simulink model "vessel_model"  (R2020a)
settings: Solver=FixedStepAuto  StartTime=0.0  StopTime=10  FixedStep=0.01  RelTol=1e-3
PreLoadFcn:
  | load("interfaces.mat");
libraries: simulink_extras x5
settings Model: Creator=thomas.evang  LastModifiedBy=thomas.evang
settings SFSimCC: CustomCodeUndefinedFunction=UseInterfaceOnly
settings RTWCC: Description=Generic Real-Time Target  RetainRTWFile=on

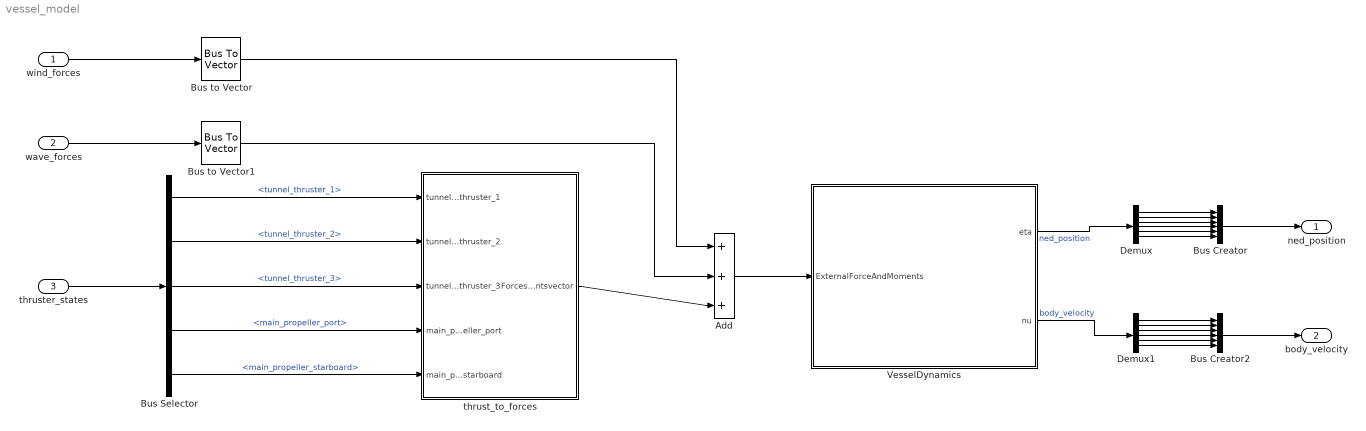
== system vessel_model ==
  wind_forces : Inport  OutDataTypeStr=Bus: force_6dof
  wave_forces : Inport  Port=2  OutDataTypeStr=Bus: force_6dof
  thruster_states : Inport  Port=3  OutDataTypeStr=Bus: thruster_states
  Add : Sum  Inputs=+++|
  Bus Creator : BusCreator  Inputs=6  OutDataTypeStr=Bus: position_6dof
      settings: InheritFromInputs=off
  Bus Creator2 : BusCreator  Inputs=6  OutDataTypeStr=Bus: velocity_6dof
      settings: InheritFromInputs=off
  Bus Selector : BusSelector  OutputSignals=tunnel_thruster_1,tunnel_thruster_2,tunnel_thruster_3,main_propeller_port,main_propeller_starboard
  Bus to Vector : BusToVector
  Bus to Vector1 : BusToVector
  Demux : Demux  Outputs=6
  Demux1 : Demux  Outputs=6
  VesselDynamics : Subsystem
  thrust_to_forces : Subsystem
  ned_position : Outport  OutDataTypeStr=Bus: position_6dof  VectorParamsAs1DForOutWhenUnconnected=off
  body_velocity : Outport  Port=2  OutDataTypeStr=Bus: velocity_6dof  VectorParamsAs1DForOutWhenUnconnected=off
  wires:
  wave_forces/1 -> Bus to Vector1/1
  wind_forces/1 -> Bus to Vector/1
  thruster_states/1 -> Bus Selector/1
  Bus Selector/1 -> thrust_to_forces/1(tunnel_thruster_1)  "<tunnel_thruster_1>"
  Bus Selector/2 -> thrust_to_forces/2(tunnel_thruster_2)  "<tunnel_thruster_2>"
  Bus Selector/3 -> thrust_to_forces/3(tunnel_thruster_3)  "<tunnel_thruster_3>"
  Bus Selector/4 -> thrust_to_forces/4(main_propeller_port)  "<main_propeller_port>"
  Bus Selector/5 -> thrust_to_forces/5(main_propeller_starboard)  "<main_propeller_starboard>"
  Bus to Vector/1 -> Add/1
  Bus to Vector1/1 -> Add/2
  VesselDynamics/1(eta) -> Demux/1  "ned_position"
  Demux/1 -> Bus Creator/1
  Demux/2 -> Bus Creator/2
  Demux/3 -> Bus Creator/3
  Demux/4 -> Bus Creator/4
  Demux/5 -> Bus Creator/5
  Demux/6 -> Bus Creator/6
  Demux1/3 -> Bus Creator2/3
  Demux1/6 -> Bus Creator2/6
  Demux1/2 -> Bus Creator2/2
  Demux1/5 -> Bus Creator2/5
  Demux1/1 -> Bus Creator2/1
  VesselDynamics/2(nu) -> Demux1/1  "body_velocity"
  Demux1/4 -> Bus Creator2/4
  Bus Creator/1 -> ned_position/1
  Bus Creator2/1 -> body_velocity/1
  thrust_to_forces/1(ForcesAndMomentsvector) -> Add/3
  Add/1 -> VesselDynamics/1(ExternalForceAndMoments)

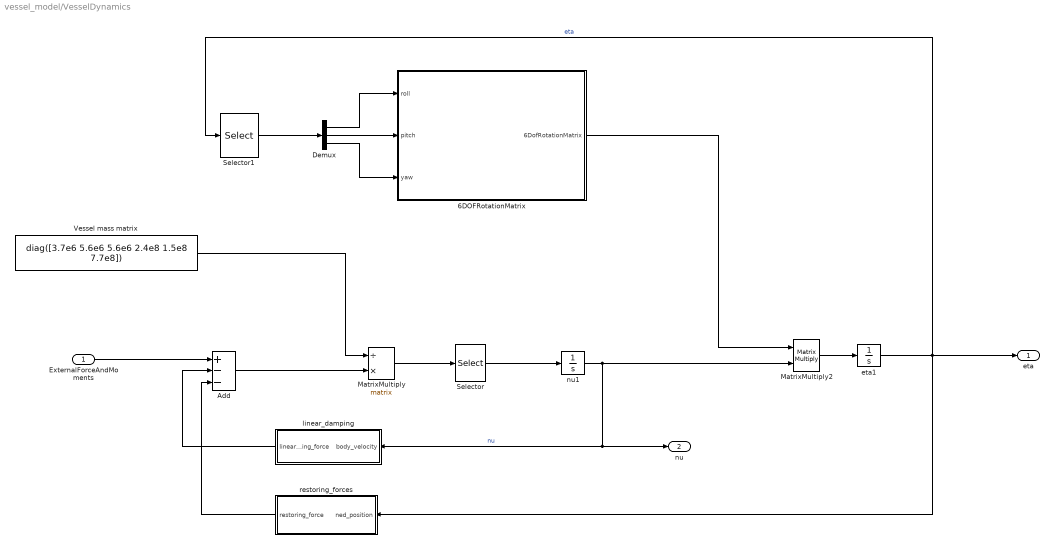
== system vessel_model/VesselDynamics ==
  ExternalForceAndMoments : Inport
  6DOFRotationMatrix : Subsystem
  Add : Sum  Inputs=+--
  Demux : Demux  Outputs=3
  MatrixMultiply : Product  Inputs=/*  Multiplication=Matrix(*)
  MatrixMultiply2 : Product  Inputs=**  Multiplication=Matrix(*)
  Selector : Selector  NumberOfDimensions=2  InputPortWidth=3  IndexOptions=Select all,Index vector (dialog)  Indices=[1 3],1  OutputSizes=1,1
  Selector1 : Selector  InputPortWidth=6  IndexOptions=Index vector (dialog)  Indices=[4 5 6]  OutputSizes=1
  Vessel mass matrix : Constant  Value=diag([3.7e6 5.6e6 5.6e6 2.4e8 1.5e8 7.7e8])
  eta1 : Integrator  InitialCondition=zeros(6,1)  ContinuousStateAttributes='nu'
  linear_damping : Subsystem
  nu1 : Integrator  InitialCondition=zeros(6,1)  ContinuousStateAttributes='eta'
  restoring_forces : Subsystem  mask{a_wp=1548, gm_t=1.5, gm_l=61, rho_w=1025, g=9.81, disp=2000*10}
      mask prompts: a_wp "Water Plane Area"; gm_t "Transverse Metacentric Height"; gm_l "Longitudal Metacentric Height"; rho_w "Density of Water"; g "Gravity"; disp "Displacement"
  eta : Outport  VectorParamsAs1DForOutWhenUnconnected=off
  nu : Outport  Port=2  VectorParamsAs1DForOutWhenUnconnected=off
  wires:
  Demux/2 -> 6DOFRotationMatrix/2(pitch)
  nu1/1 -> MatrixMultiply2/2, linear_damping/1(body_velocity), nu/1  "nu"
  Vessel mass matrix/1 -> MatrixMultiply/1
  Demux/1 -> 6DOFRotationMatrix/1(roll)
  Selector1/1 -> Demux/1
  Demux/3 -> 6DOFRotationMatrix/3(yaw)
  Add/1 -> MatrixMultiply/2
  MatrixMultiply/1 -> Selector/1
  Selector/1 -> nu1/1
  6DOFRotationMatrix/1(6DofRotationMatrix) -> MatrixMultiply2/1
  eta1/1 -> eta/1, restoring_forces/1(ned_position), Selector1/1  "eta"
  ExternalForceAndMoments/1 -> Add/1
  MatrixMultiply2/1 -> eta1/1
  restoring_forces/1(restoring_force) -> Add/3
  linear_damping/1(linear_damping_force) -> Add/2

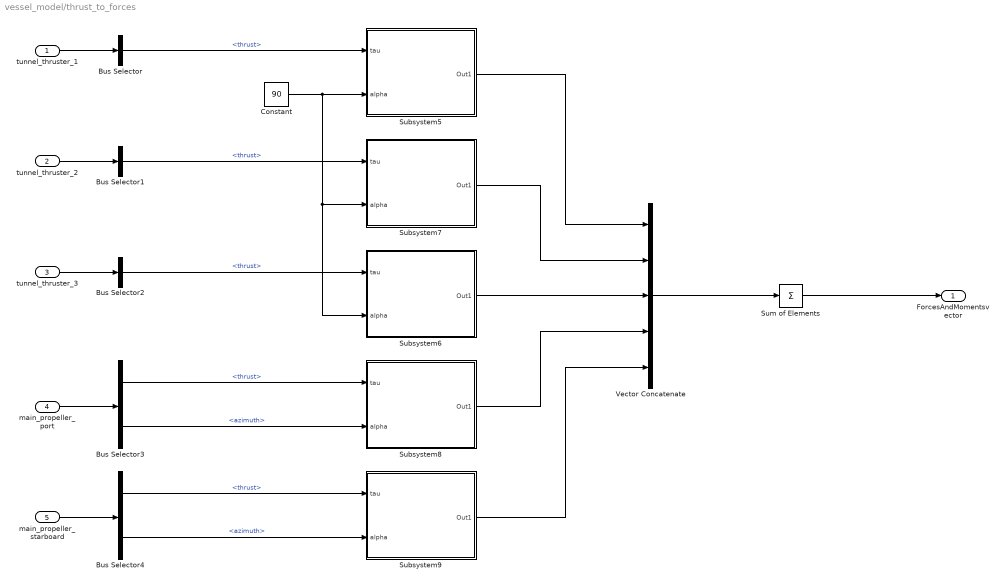
== system vessel_model/thrust_to_forces ==
  tunnel_thruster_1 : Inport  OutDataTypeStr=Bus: tunnel_thruster
  tunnel_thruster_2 : Inport  Port=2  OutDataTypeStr=Bus: tunnel_thruster
  tunnel_thruster_3 : Inport  Port=3  OutDataTypeStr=Bus: tunnel_thruster
  main_propeller_port : Inport  Port=4  OutDataTypeStr=Bus: azimuth_thruster
  main_propeller_starboard : Inport  Port=5  OutDataTypeStr=Bus: azimuth_thruster
  Bus Selector : BusSelector  OutputSignals=thrust
  Bus Selector1 : BusSelector  OutputSignals=thrust
  Bus Selector2 : BusSelector  OutputSignals=thrust
  Bus Selector3 : BusSelector  OutputSignals=thrust,azimuth
  Bus Selector4 : BusSelector  OutputSignals=thrust,azimuth
  Constant : Constant  Value=90
  Subsystem5 : Subsystem  mask{x=31.25, y=0, z=2.1}
  Subsystem6 : Subsystem  mask{x=24.75, y=0, z=1.9}
  Subsystem7 : Subsystem  mask{x=28.9, y=0, z=1.9}
  Subsystem8 : Subsystem  mask{x=-36.45, y=-4, z=1.415}
  Subsystem9 : Subsystem  mask{x=-36.45, y=4, z=1.415}
  Sum of Elements : Sum  Inputs=+  CollapseMode=Specified dimension  CollapseDim=2
  Vector Concatenate : Concatenate  NumInputs=5  Mode=Multidimensional array  ConcatenateDimension=2
  ForcesAndMomentsvector : Outport  VectorParamsAs1DForOutWhenUnconnected=off
  wires:
  Constant/1 -> Subsystem5/2(alpha), Subsystem6/2(alpha), Subsystem7/2(alpha)
  Subsystem9/1(Out1) -> Vector Concatenate/5
  Subsystem5/1(Out1) -> Vector Concatenate/1
  Vector Concatenate/1 -> Sum of Elements/1
  Subsystem8/1(Out1) -> Vector Concatenate/4
  Subsystem7/1(Out1) -> Vector Concatenate/2
  Subsystem6/1(Out1) -> Vector Concatenate/3
  tunnel_thruster_1/1 -> Bus Selector/1
  Bus Selector1/1 -> Subsystem7/1(tau)  "<thrust>"
  tunnel_thruster_2/1 -> Bus Selector1/1
  tunnel_thruster_3/1 -> Bus Selector2/1
  Bus Selector2/1 -> Subsystem6/1(tau)  "<thrust>"
  main_propeller_port/1 -> Bus Selector3/1
  Bus Selector3/1 -> Subsystem8/1(tau)  "<thrust>"
  Bus Selector3/2 -> Subsystem8/2(alpha)  "<azimuth>"
  Bus Selector4/2 -> Subsystem9/2(alpha)  "<azimuth>"
  Bus Selector4/1 -> Subsystem9/1(tau)  "<thrust>"
  main_propeller_starboard/1 -> Bus Selector4/1
  Bus Selector/1 -> Subsystem5/1(tau)  "<thrust>"
  Sum of Elements/1 -> ForcesAndMomentsvector/1

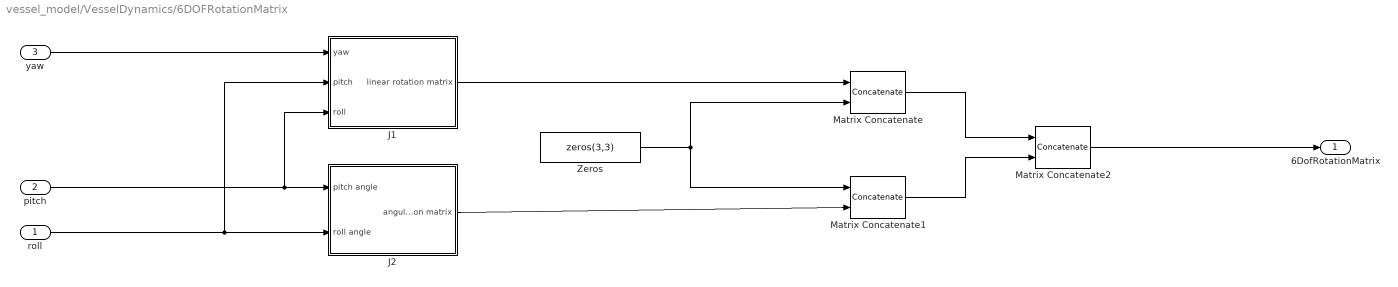
== system vessel_model/VesselDynamics/6DOFRotationMatrix ==
  roll : Inport
  pitch : Inport  Port=2
  yaw : Inport  Port=3
  J1 : Subsystem
  J2 : Subsystem
  Matrix Concatenate : Concatenate  Mode=Multidimensional array
  Matrix Concatenate1 : Concatenate  Mode=Multidimensional array
  Matrix Concatenate2 : Concatenate  Mode=Multidimensional array  ConcatenateDimension=2
  Zeros : Constant  Value=zeros(3,3)
  6DofRotationMatrix : Outport  VectorParamsAs1DForOutWhenUnconnected=off
  wires:
  pitch/1 -> J1/3(roll), J2/1(pitch angle)
  roll/1 -> J2/2(roll angle), J1/2(pitch)
  Zeros/1 -> Matrix Concatenate/2, Matrix Concatenate1/1
  Matrix Concatenate1/1 -> Matrix Concatenate2/2
  Matrix Concatenate/1 -> Matrix Concatenate2/1
  Matrix Concatenate2/1 -> 6DofRotationMatrix/1
  J2/1(angular rotation matrix) -> Matrix Concatenate1/2
  yaw/1 -> J1/1(yaw)
  J1/1(linear rotation matrix) -> Matrix Concatenate/1

== system vessel_model/VesselDynamics/linear_damping ==
  body_velocity : Inport
  DampingForces : Product  Multiplication=Matrix(*)
  Vessel Damping Matrix : Constant  Value=diag([7.8e3 4.3e4 5.4e6 1.6e9 2.6e9 1.9e7])
  linear_damping_force : Outport  VectorParamsAs1DForOutWhenUnconnected=off
  wires:
  Vessel Damping Matrix/1 -> DampingForces/1
  body_velocity/1 -> DampingForces/2
  DampingForces/1 -> linear_damping_force/1

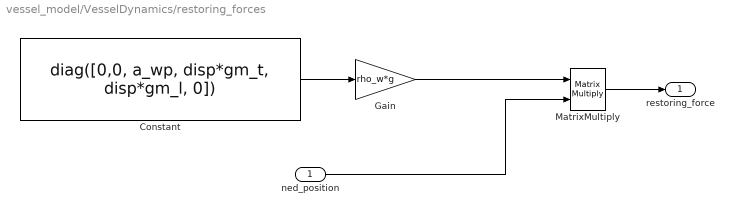
== system vessel_model/VesselDynamics/restoring_forces ==
  ned_position : Inport  PortDimensions=6
  Constant : Constant  Value=diag([0,0, a_wp, disp*gm_t, disp*gm_l, 0])
  Gain : Gain  Gain=rho_w*g
  MatrixMultiply : Product  Multiplication=Matrix(*)
  restoring_force : Outport  VectorParamsAs1DForOutWhenUnconnected=off
  wires:
  Constant/1 -> Gain/1
  Gain/1 -> MatrixMultiply/1
  ned_position/1 -> MatrixMultiply/2
  MatrixMultiply/1 -> restoring_force/1

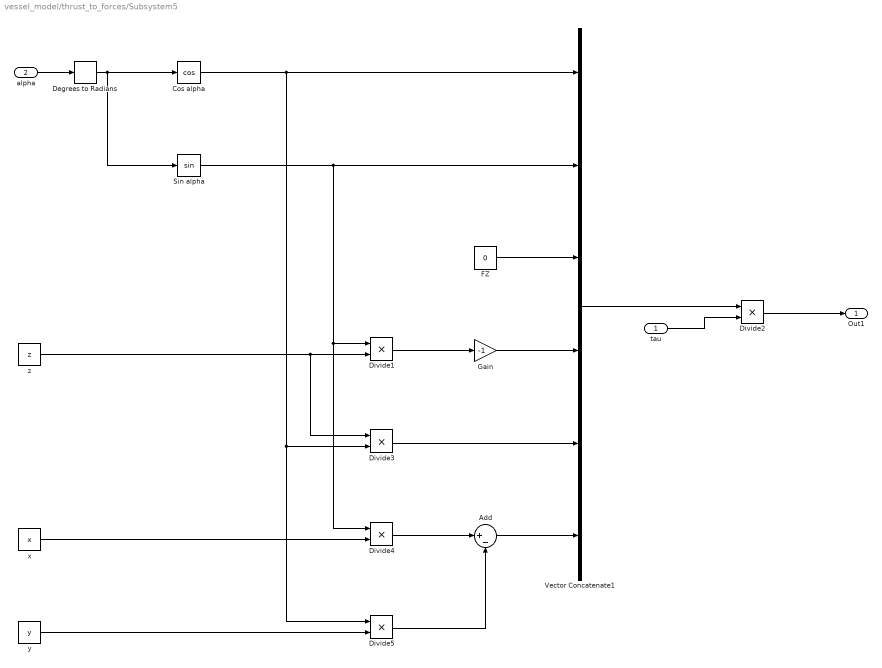
== system vessel_model/thrust_to_forces/Subsystem5 ==
  tau : Inport  OutDataTypeStr=double  PortDimensions=1
  alpha : Inport  Port=2  OutDataTypeStr=double  PortDimensions=1
  Add : Sum  Inputs=|+-
  Cos alpha : Trigonometry  Operator=cos
  Degrees to Radians : simulink_extras/Transformations/Degrees to Radians
  Divide{1..5} (5 alike) : Product
  FZ : Constant  Value=0
  Gain : Gain  Gain=-1
  Sin alpha : Trigonometry
  Vector Concatenate1 : Concatenate  NumInputs=6
  x : Constant  Value=x
  y : Constant  Value=y
  z : Constant  Value=z
  Out1 : Outport  OutDataTypeStr=double  PortDimensions=6  VectorParamsAs1DForOutWhenUnconnected=off
  wires:
  Sin alpha/1 -> Divide4/1, Divide1/1, Vector Concatenate1/2
  tau/1 -> Divide2/2
  y/1 -> Divide5/2
  Degrees to Radians/1 -> Sin alpha/1, Cos alpha/1
  Gain/1 -> Vector Concatenate1/4
  z/1 -> Divide1/2, Divide3/1
  Cos alpha/1 -> Divide5/1, Divide3/2, Vector Concatenate1/1
  Divide1/1 -> Gain/1
  Divide5/1 -> Add/2
  Divide2/1 -> Out1/1
  Divide3/1 -> Vector Concatenate1/5
  x/1 -> Divide4/2
  Divide4/1 -> Add/1
  Add/1 -> Vector Concatenate1/6
  FZ/1 -> Vector Concatenate1/3
  Vector Concatenate1/1 -> Divide2/1
  alpha/1 -> Degrees to Radians/1

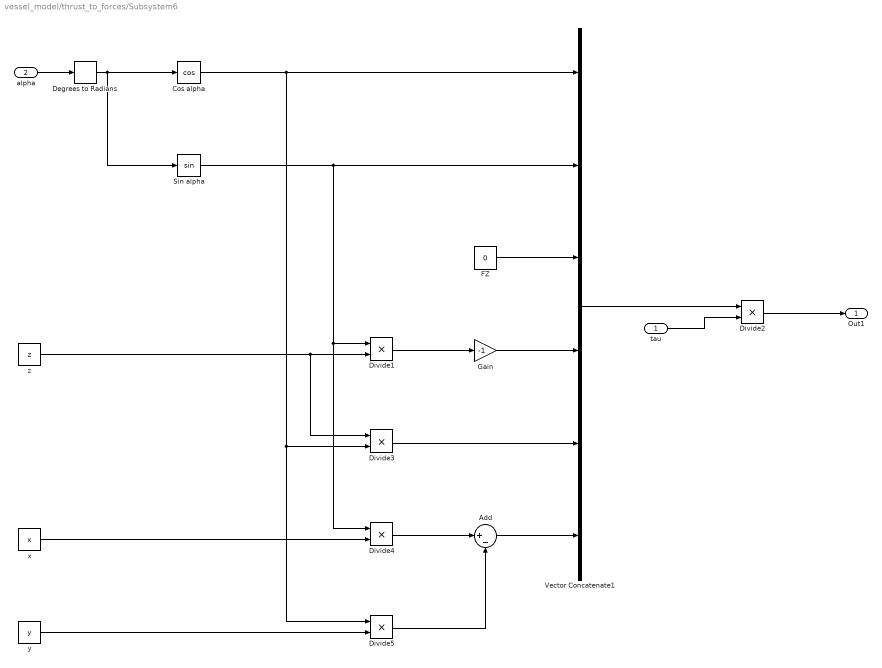
== system vessel_model/thrust_to_forces/Subsystem6 ==
  tau : Inport  OutDataTypeStr=double  PortDimensions=1
  alpha : Inport  Port=2  OutDataTypeStr=double  PortDimensions=1
  Add : Sum  Inputs=|+-
  Cos alpha : Trigonometry  Operator=cos
  Degrees to Radians : simulink_extras/Transformations/Degrees to Radians
  Divide{1..5} (5 alike) : Product
  FZ : Constant  Value=0
  Gain : Gain  Gain=-1
  Sin alpha : Trigonometry
  Vector Concatenate1 : Concatenate  NumInputs=6
  x : Constant  Value=x
  y : Constant  Value=y
  z : Constant  Value=z
  Out1 : Outport  OutDataTypeStr=double  PortDimensions=6  VectorParamsAs1DForOutWhenUnconnected=off
  wires:
  alpha/1 -> Degrees to Radians/1
  Vector Concatenate1/1 -> Divide2/1
  FZ/1 -> Vector Concatenate1/3
  Add/1 -> Vector Concatenate1/6
  Divide4/1 -> Add/1
  x/1 -> Divide4/2
  Divide3/1 -> Vector Concatenate1/5
  Divide2/1 -> Out1/1
  Divide5/1 -> Add/2
  Divide1/1 -> Gain/1
  Cos alpha/1 -> Vector Concatenate1/1, Divide3/2, Divide5/1
  z/1 -> Divide3/1, Divide1/2
  Gain/1 -> Vector Concatenate1/4
  Degrees to Radians/1 -> Cos alpha/1, Sin alpha/1
  y/1 -> Divide5/2
  tau/1 -> Divide2/2
  Sin alpha/1 -> Vector Concatenate1/2, Divide1/1, Divide4/1

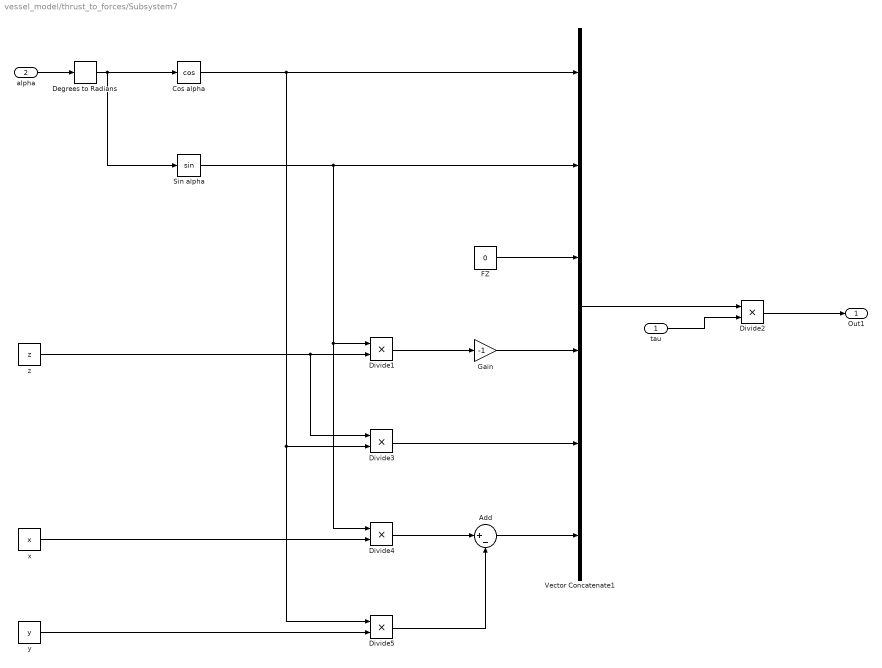
== system vessel_model/thrust_to_forces/Subsystem7 ==
  tau : Inport  OutDataTypeStr=double  PortDimensions=1
  alpha : Inport  Port=2  OutDataTypeStr=double  PortDimensions=1
  Add : Sum  Inputs=|+-
  Cos alpha : Trigonometry  Operator=cos
  Degrees to Radians : simulink_extras/Transformations/Degrees to Radians
  Divide{1..5} (5 alike) : Product
  FZ : Constant  Value=0
  Gain : Gain  Gain=-1
  Sin alpha : Trigonometry
  Vector Concatenate1 : Concatenate  NumInputs=6
  x : Constant  Value=x
  y : Constant  Value=y
  z : Constant  Value=z
  Out1 : Outport  OutDataTypeStr=double  PortDimensions=6  VectorParamsAs1DForOutWhenUnconnected=off
  wires:
  alpha/1 -> Degrees to Radians/1
  Vector Concatenate1/1 -> Divide2/1
  FZ/1 -> Vector Concatenate1/3
  Add/1 -> Vector Concatenate1/6
  Divide4/1 -> Add/1
  x/1 -> Divide4/2
  Divide3/1 -> Vector Concatenate1/5
  Divide2/1 -> Out1/1
  Divide5/1 -> Add/2
  Divide1/1 -> Gain/1
  Cos alpha/1 -> Vector Concatenate1/1, Divide3/2, Divide5/1
  z/1 -> Divide3/1, Divide1/2
  Gain/1 -> Vector Concatenate1/4
  Degrees to Radians/1 -> Cos alpha/1, Sin alpha/1
  y/1 -> Divide5/2
  tau/1 -> Divide2/2
  Sin alpha/1 -> Vector Concatenate1/2, Divide1/1, Divide4/1

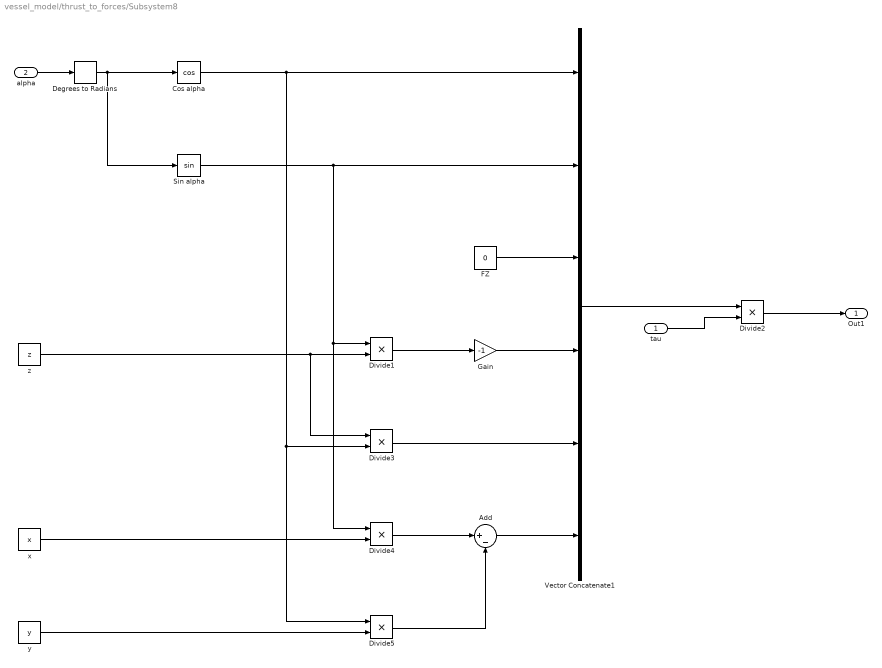
== system vessel_model/thrust_to_forces/Subsystem8 ==
  tau : Inport  OutDataTypeStr=double  PortDimensions=1
  alpha : Inport  Port=2  OutDataTypeStr=double  PortDimensions=1
  Add : Sum  Inputs=|+-
  Cos alpha : Trigonometry  Operator=cos
  Degrees to Radians : simulink_extras/Transformations/Degrees to Radians
  Divide{1..5} (5 alike) : Product
  FZ : Constant  Value=0
  Gain : Gain  Gain=-1
  Sin alpha : Trigonometry
  Vector Concatenate1 : Concatenate  NumInputs=6
  x : Constant  Value=x
  y : Constant  Value=y
  z : Constant  Value=z
  Out1 : Outport  OutDataTypeStr=double  PortDimensions=6  VectorParamsAs1DForOutWhenUnconnected=off
  wires:
  Sin alpha/1 -> Divide4/1, Divide1/1, Vector Concatenate1/2
  tau/1 -> Divide2/2
  y/1 -> Divide5/2
  Degrees to Radians/1 -> Sin alpha/1, Cos alpha/1
  Gain/1 -> Vector Concatenate1/4
  z/1 -> Divide1/2, Divide3/1
  Cos alpha/1 -> Divide5/1, Divide3/2, Vector Concatenate1/1
  Divide1/1 -> Gain/1
  Divide5/1 -> Add/2
  Divide2/1 -> Out1/1
  Divide3/1 -> Vector Concatenate1/5
  x/1 -> Divide4/2
  Divide4/1 -> Add/1
  Add/1 -> Vector Concatenate1/6
  FZ/1 -> Vector Concatenate1/3
  Vector Concatenate1/1 -> Divide2/1
  alpha/1 -> Degrees to Radians/1

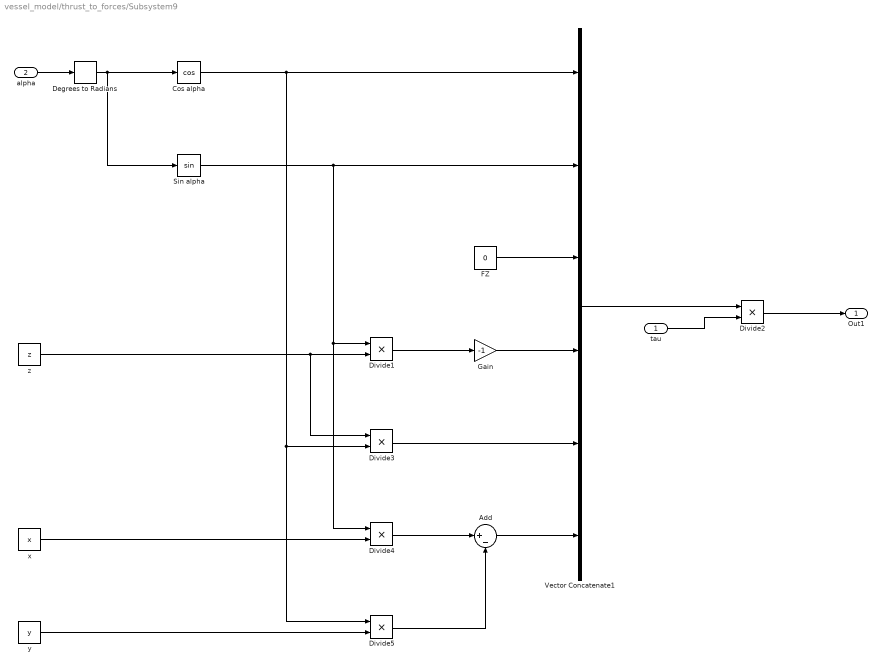
== system vessel_model/thrust_to_forces/Subsystem9 ==
  tau : Inport  OutDataTypeStr=double  PortDimensions=1
  alpha : Inport  Port=2  OutDataTypeStr=double  PortDimensions=1
  Add : Sum  Inputs=|+-
  Cos alpha : Trigonometry  Operator=cos
  Degrees to Radians : simulink_extras/Transformations/Degrees to Radians
  Divide{1..5} (5 alike) : Product
  FZ : Constant  Value=0
  Gain : Gain  Gain=-1
  Sin alpha : Trigonometry
  Vector Concatenate1 : Concatenate  NumInputs=6
  x : Constant  Value=x
  y : Constant  Value=y
  z : Constant  Value=z
  Out1 : Outport  OutDataTypeStr=double  PortDimensions=6  VectorParamsAs1DForOutWhenUnconnected=off
  wires:
  alpha/1 -> Degrees to Radians/1
  Vector Concatenate1/1 -> Divide2/1
  FZ/1 -> Vector Concatenate1/3
  Add/1 -> Vector Concatenate1/6
  Divide4/1 -> Add/1
  x/1 -> Divide4/2
  Divide3/1 -> Vector Concatenate1/5
  Divide2/1 -> Out1/1
  Divide5/1 -> Add/2
  Divide1/1 -> Gain/1
  Cos alpha/1 -> Vector Concatenate1/1, Divide3/2, Divide5/1
  z/1 -> Divide3/1, Divide1/2
  Gain/1 -> Vector Concatenate1/4
  Degrees to Radians/1 -> Cos alpha/1, Sin alpha/1
  y/1 -> Divide5/2
  tau/1 -> Divide2/2
  Sin alpha/1 -> Vector Concatenate1/2, Divide1/1, Divide4/1

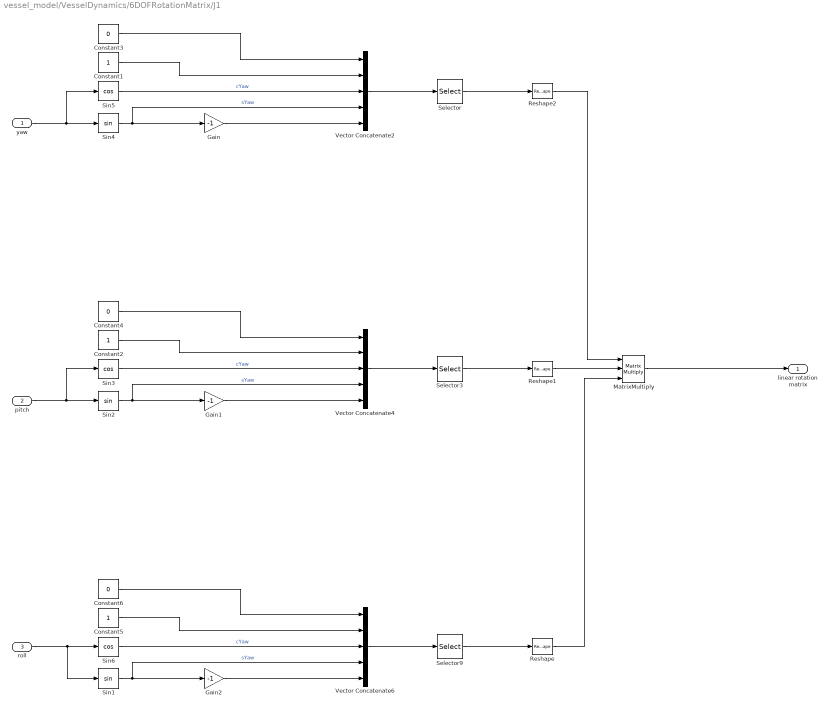
== system vessel_model/VesselDynamics/6DOFRotationMatrix/J1 ==
  yaw : Inport
  pitch : Inport  Port=2
  roll : Inport  Port=3
  Constant1 : Constant
  Constant2 : Constant
  Constant3 : Constant  Value=0
  Constant4 : Constant  Value=0
  Constant5 : Constant
  Constant6 : Constant  Value=0
  Gain : Gain  Gain=-1
  Gain1 : Gain  Gain=-1
  Gain2 : Gain  Gain=-1
  MatrixMultiply : Product  Inputs=3  Multiplication=Matrix(*)
  Reshape : Reshape  OutputDimensionality=Customize  OutputDimensions=[3,3]
  Reshape1 : Reshape  OutputDimensionality=Customize  OutputDimensions=[3,3]
  Reshape2 : Reshape  OutputDimensionality=Customize  OutputDimensions=[3,3]
  Selector : Selector  InputPortWidth=5  IndexOptions=Index vector (dialog)  Indices=[3 4 1 5 3 1 1 1 2]  OutputSizes=1
  Selector3 : Selector  InputPortWidth=5  IndexOptions=Index vector (dialog)  Indices=[3 1 5 1 2 1 4 1 3]  OutputSizes=1
  Selector9 : Selector  InputPortWidth=5  IndexOptions=Index vector (dialog)  Indices=[2 1 1 1 3 4 1 5 3]  OutputSizes=1
  Sin1 : Trigonometry
  Sin2 : Trigonometry
  Sin3 : Trigonometry  Operator=cos
  Sin4 : Trigonometry
  Sin5 : Trigonometry  Operator=cos
  Sin6 : Trigonometry  Operator=cos
  Vector Concatenate2 : Concatenate  NumInputs=5
  Vector Concatenate4 : Concatenate  NumInputs=5
  Vector Concatenate6 : Concatenate  NumInputs=5
  linear rotation matrix : Outport  VectorParamsAs1DForOutWhenUnconnected=off
  wires:
  pitch/1 -> Sin3/1, Sin2/1
  Constant6/1 -> Vector Concatenate6/1
  Sin3/1 -> Vector Concatenate4/3  "cYaw"
  Constant5/1 -> Vector Concatenate6/2
  MatrixMultiply/1 -> linear rotation matrix/1
  Sin1/1 -> Vector Concatenate6/4, Gain2/1  "sYaw"
  Selector/1 -> Reshape2/1
  yaw/1 -> Sin5/1, Sin4/1
  Reshape/1 -> MatrixMultiply/3
  Sin2/1 -> Gain1/1, Vector Concatenate4/4  "sYaw"
  Sin6/1 -> Vector Concatenate6/3  "cYaw"
  Sin4/1 -> Vector Concatenate2/4, Gain/1  "sYaw"
  Selector3/1 -> Reshape1/1
  Reshape1/1 -> MatrixMultiply/2
  Gain2/1 -> Vector Concatenate6/5
  Vector Concatenate6/1 -> Selector9/1
  Selector9/1 -> Reshape/1
  Gain/1 -> Vector Concatenate2/5
  Reshape2/1 -> MatrixMultiply/1
  Vector Concatenate2/1 -> Selector/1
  Vector Concatenate4/1 -> Selector3/1
  Constant1/1 -> Vector Concatenate2/2
  roll/1 -> Sin1/1, Sin6/1
  Gain1/1 -> Vector Concatenate4/5
  Constant4/1 -> Vector Concatenate4/1
  Constant2/1 -> Vector Concatenate4/2
  Constant3/1 -> Vector Concatenate2/1
  Sin5/1 -> Vector Concatenate2/3  "cYaw"

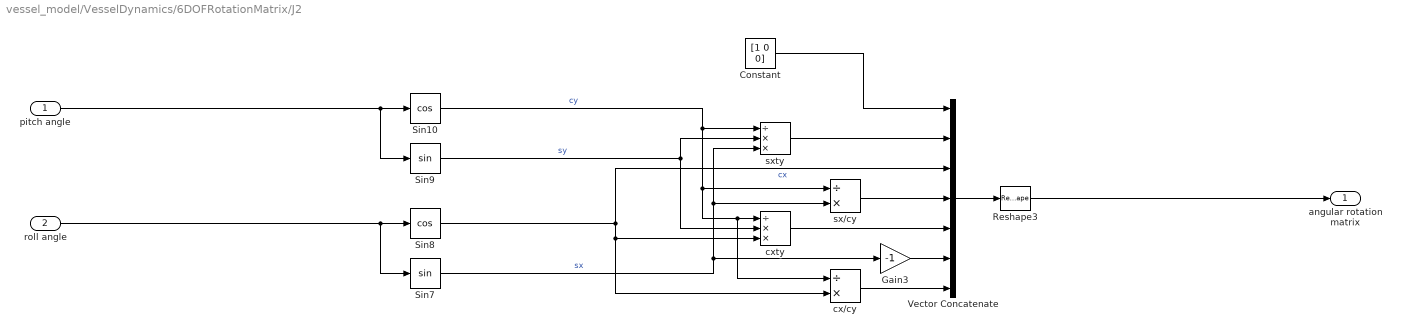
== system vessel_model/VesselDynamics/6DOFRotationMatrix/J2 ==
  pitch angle : Inport
  roll angle : Inport  Port=2
  Constant : Constant  Value=[1 0 0]
  Gain3 : Gain  Gain=-1
  Reshape3 : Reshape  OutputDimensionality=Customize  OutputDimensions=[3,3]
  Sin10 : Trigonometry  Operator=cos
  Sin7 : Trigonometry
  Sin8 : Trigonometry  Operator=cos
  Sin9 : Trigonometry
  Vector Concatenate : Concatenate  NumInputs=7
  cx/cy : Product  Inputs=/*
  cxty : Product  Inputs=/**
  sx/cy : Product  Inputs=/*
  sxty : Product  Inputs=/**
  angular rotation matrix : Outport  VectorParamsAs1DForOutWhenUnconnected=off
  wires:
  Sin7/1 -> sxty/3, sx/cy/2, Gain3/1  "sx"
  pitch angle/1 -> Sin9/1, Sin10/1
  sxty/1 -> Vector Concatenate/2
  Sin9/1 -> cxty/2, sxty/2  "sy"
  roll angle/1 -> Sin7/1, Sin8/1
  cxty/1 -> Vector Concatenate/5
  Sin8/1 -> cx/cy/2, cxty/3, Vector Concatenate/3  "cx"
  sx/cy/1 -> Vector Concatenate/4
  cx/cy/1 -> Vector Concatenate/7
  Vector Concatenate/1 -> Reshape3/1
  Sin10/1 -> sx/cy/1, cx/cy/1, cxty/1, sxty/1  "cy"
  Constant/1 -> Vector Concatenate/1
  Gain3/1 -> Vector Concatenate/6
  Reshape3/1 -> angular rotation matrix/1
